simulink model "FuzzyConditioner"  (R2021b)
settings: Solver=ode45  StartTime=0.0  StopTime=100.0  RelTol=1e-3  EnableMultiTasking=on
libraries: fuzblock x2
settings Model: Creator=Aaa  LastModifiedBy=User
settings SolverCC: AlgebraicLoopSolver=TrustRegion
settings DataIOCC: LimitDataPoints=on  SaveFormat=Array  ReturnWorkspaceOutputs=off
settings OptimizationCC: LifeSpan=inf
settings DebuggingCC: SolverPrmCheckMsg=warning  SFUnexpectedBacktrackingDiag=warning  SFNoUnconditionalDefaultTransitionDiag=warning  SFExecutionAtInitializationDiag=none  SFMachineParentedDataDiag=warning  ArithmeticOperatorsInVariantConditions=warning
settings HardwareCC: ProdBitPerPointer=32  ProdBitPerSizeT=32  ProdBitPerPtrDiffT=32  ProdLargestAtomicFloat=None  ProdIntDivRoundTo=Undefined  ProdEndianess=Unspecified  ProdWordSize=32  ProdHWDeviceType=32-bit Generic
settings ModelReferenceCC: PropagateSignalLabelsOutOfModel=off
settings SFSimCC: SimUseLocalCustomCode=off  CustomCodeUndefinedFunction=UseInterfaceOnly
settings RTWCC: RTWUseLocalCustomCode=off
settings CodeAppCC: StateflowObjectComments=on
settings GRTTargetCC: TargetLangStandard=C89/C90 (ANSI)
settings ConfigComp: CovMetricSettings=dw  CovSaveCumulativeToWorkspaceVar=on  CovSaveSingleToWorkspaceVar=on  CovExternalEMLEnable=off  CovSFcnEnable=off

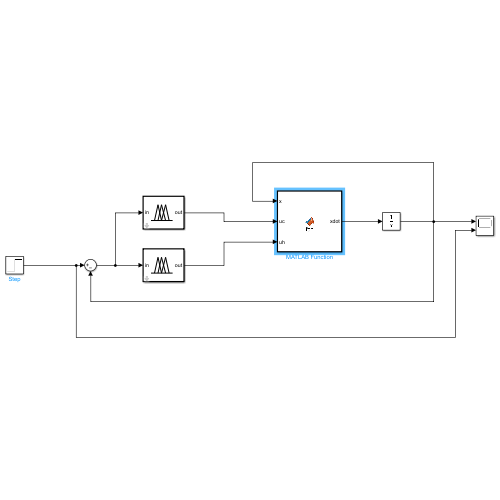
[thumbnail: Simulink's stored preview of the top-level diagram]
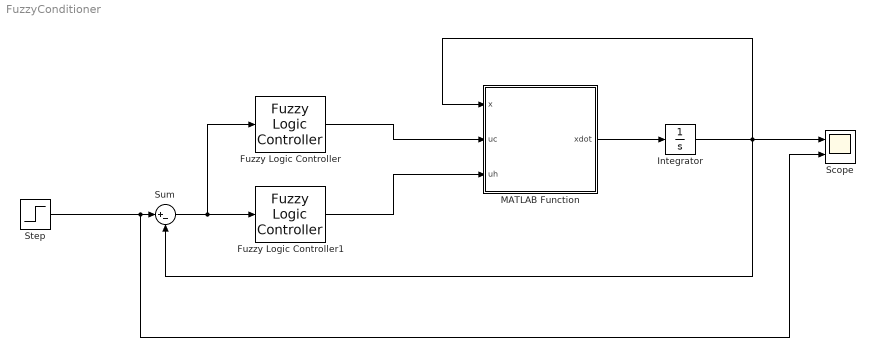
== system FuzzyConditioner ==
  Fuzzy Logic Controller : fuzblock/Fuzzy Logic  Controller  FIS='Cooler.fis'  OutputSampleNumber=101  DataType=double  FuzzifiedInputs=off  RuleFiringStrengths=off  RuleOutputs=off  AggregatedOutputs=off  SimulateUsing=Interpreted execution  OutOfRangeInputValueMessage=warning  NoRuleFiredMessage=warning  EmptyOutputFuzzySetMessage=warning
  Fuzzy Logic Controller1 : fuzblock/Fuzzy Logic  Controller  FIS='Heater.fis'  OutputSampleNumber=101  DataType=double  FuzzifiedInputs=off  RuleFiringStrengths=off  RuleOutputs=off  AggregatedOutputs=off  SimulateUsing=Interpreted execution  OutOfRangeInputValueMessage=warning  NoRuleFiredMessage=warning  EmptyOutputFuzzySetMessage=warning
  Integrator : Integrator
  MATLAB Function : MATLAB Function  TreatAsAtomicUnit=on
  Scope : Scope  NumInputPorts=2
  Step : Step  After=16  SampleTime=0
  Sum : Sum  Inputs=|+-
  wires:
  Integrator/1 -> Sum/2, MATLAB Function/1(x), Scope/1
  Step/1 -> Scope/2, Sum/1
  Sum/1 -> Fuzzy Logic Controller/1, Fuzzy Logic Controller1/1
  MATLAB Function/1(xdot) -> Integrator/1
  Fuzzy Logic Controller/1 -> MATLAB Function/2(uc)
  Fuzzy Logic Controller1/1 -> MATLAB Function/3(uh)

== matlab function FuzzyConditioner/MATLAB Function ==
  data: x input; xdot output; uc input; uh input
function xdot = fcn(x,uc,uh)
xdot = -(x-20) - 2*uc + 2*uh;
